simulink model "camera_model"  (R2020a)
settings: Solver=FixedStepDiscrete  StartTime=0.0  StopTime=10000-1  FixedStep=1  RelTol=1e-3
values from neighbouring files (symbols this model uses):
  focal_length = 0.05    [initialization_camera.m]
  FOV_M = 15    [initialization_camera.m]
  FOV_N = 30    [initialization_camera.m]
  pattern_dim = pattern_dim_v(cont_pd)    [initialization_camera.m]
settings Model: Creator=lu  LastModifiedBy=utente
settings DataIOCC: SaveTime=off  ReturnWorkspaceOutputs=off
settings DebuggingCC: ArithmeticOperatorsInVariantConditions=warning
settings SFSimCC: CustomCodeUndefinedFunction=UseInterfaceOnly

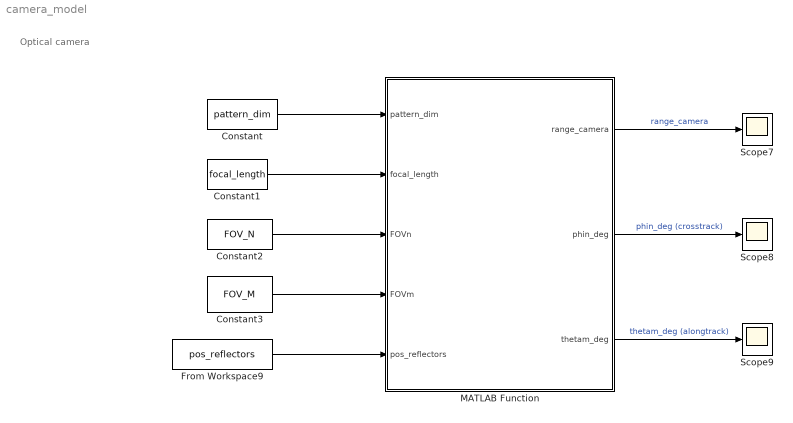
== system camera_model ==
  note: Optical camera
  Constant : Constant  Value=pattern_dim
  Constant1 : Constant  Value=focal_length
  Constant2 : Constant  Value=FOV_N
  Constant3 : Constant  Value=FOV_M
  From Workspace9 : FromWorkspace  VariableName=pos_reflectors
  MATLAB Function : MATLAB Function  TreatAsAtomicUnit=on
  Scope7 : Scope
  Scope8 : Scope
  Scope9 : Scope
  wires:
  MATLAB Function/1(range_camera) -> Scope7/1  "range_camera"
  MATLAB Function/3(thetam_deg) -> Scope9/1  "thetam_deg (alongtrack)"
  MATLAB Function/2(phin_deg) -> Scope8/1  "phin_deg (crosstrack)"
  Constant/1 -> MATLAB Function/1(pattern_dim)
  From Workspace9/1 -> MATLAB Function/5(pos_reflectors)
  Constant1/1 -> MATLAB Function/2(focal_length)
  Constant2/1 -> MATLAB Function/3(FOVn)
  Constant3/1 -> MATLAB Function/4(FOVm)

== matlab function camera_model/MATLAB Function ==
  data: pattern_dim input; range_camera output; focal_length input; FOVn input; FOVm input; pos_reflectors input; phin_deg output; thetam_deg output
function [range_camera,phin_deg,thetam_deg] = fcn(pattern_dim,focal_length,FOVn,FOVm,pos_reflectors)

pos_xmin=1;
pos_xmax=1;
pos_ymin=1;
pos_ymax=1;

% focal plane dimensions
xfp=focal_length*tand(FOVn); % [m]
yfp=focal_length*tand(FOVm); % [m]

x_reflectors=pos_reflectors(1:2:end);
y_reflectors=pos_reflectors(2:2:end);

% ELLIPSE CENTRE AND AXES DETERMINATION
xmin=min(x_reflectors);
xmax=max(x_reflectors);
ymin=min(y_reflectors);
ymax=max(y_reflectors);

xcentre=(xmax+xmin)/2; %centre coordinates
ycentre=(ymax+ymin)/2;

for i=1:4
    if x_reflectors(i)==xmin
        pos_xmin=i;
    end
    if x_reflectors(i)==xmax
        pos_xmax=i;
    end
    if y_reflectors(i)==ymin
        pos_ymin=i;    
    end
    if y_reflectors(i)==ymax
        pos_ymax=i;    
    end
end

a1=sqrt((x_reflectors(pos_xmin)-x_reflectors(pos_xmax))^2+(y_reflectors(pos_xmin)-y_reflectors(pos_xmax))^2);
a2=sqrt((x_reflectors(pos_ymin)-x_reflectors(pos_ymax))^2+(y_reflectors(pos_ymin)-pos_reflectors(pos_ymax))^2);

amax=max(a1,a2); % major axis

% RANGE DETERMINATION
range_camera=pattern_dim*focal_length/amax;

% LOS DETERMINATION
phin=FOVn*xcentre/xfp; %rad
thetam=FOVm*ycentre/yfp; %rad

phin_deg=phin*180/pi; % deg
thetam_deg=thetam*180/pi; % deg
